simulink model "InvPendu_RBF"  (R2020b)
settings: Solver=VariableStepAuto  StartTime=0.0  StopTime=50  RelTol=1e-3
settings Model: Creator=lenovo  LastModifiedBy=lenovo

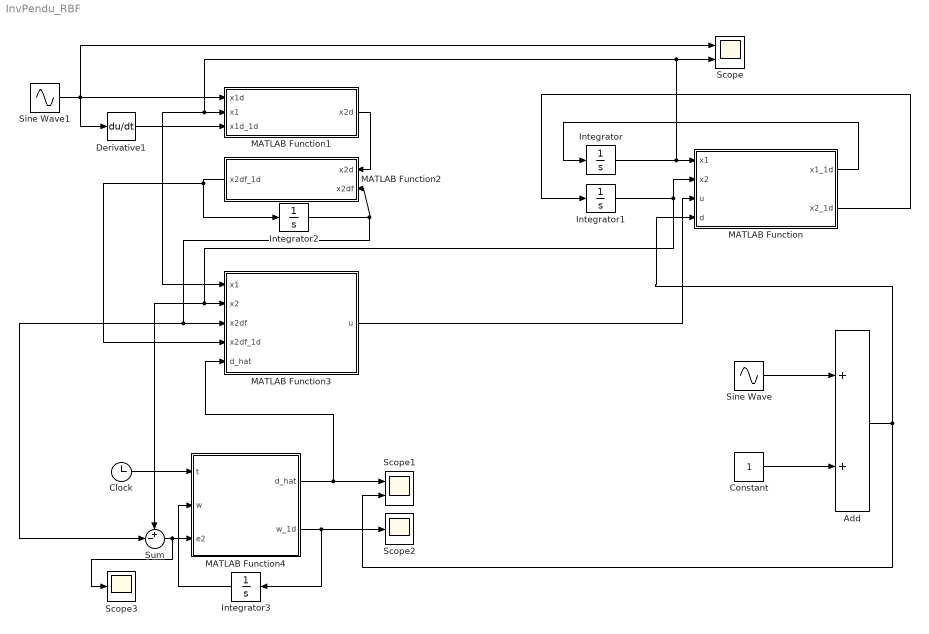
== system InvPendu_RBF ==
  Add : Sum
  Clock : Clock
  Constant : Constant
  Derivative1 : Derivative
  Integrator{,1..3} (4 alike) : Integrator
  MATLAB Function : MATLAB Function  TreatAsAtomicUnit=on
  MATLAB Function1 : MATLAB Function  TreatAsAtomicUnit=on
  MATLAB Function2 : MATLAB Function  TreatAsAtomicUnit=on
  MATLAB Function3 : MATLAB Function  TreatAsAtomicUnit=on
  MATLAB Function4 : MATLAB Function  TreatAsAtomicUnit=on
  Scope : Scope  NumInputPorts=2
  Scope1 : Scope  NumInputPorts=2
  Scope2 : Scope
  Scope3 : Scope
  Sine Wave : Sin  SampleTime=0
  Sine Wave1 : Sin  SampleTime=0
  Sum : Sum  Inputs=+-|
  wires:
  MATLAB Function/1(x1_1d) -> Integrator/1
  Integrator/1 -> Scope/2, MATLAB Function3/1(x1), MATLAB Function1/2(x1), MATLAB Function/1(x1)
  MATLAB Function/2(x2_1d) -> Integrator1/1
  Add/1 -> MATLAB Function/4(d), Scope1/2
  MATLAB Function3/1(u) -> MATLAB Function/3(u)
  Constant/1 -> Add/2
  MATLAB Function2/1(x2df_1d) -> MATLAB Function3/4(x2df_1d), Integrator2/1
  Integrator2/1 -> MATLAB Function3/3(x2df), Sum/2, MATLAB Function2/2(x2df)
  Derivative1/1 -> MATLAB Function1/3(x1d_1d)
  MATLAB Function1/1(x2d) -> MATLAB Function2/1(x2d)
  Sine Wave1/1 -> Derivative1/1, Scope/1, MATLAB Function1/1(x1d)
  Sine Wave/1 -> Add/1
  MATLAB Function4/1(d_hat) -> MATLAB Function3/5(d_hat), Scope1/1
  Integrator1/1 -> Sum/1, MATLAB Function3/2(x2), MATLAB Function/2(x2)
  Clock/1 -> MATLAB Function4/1(t)
  MATLAB Function4/2(w_1d) -> Scope2/1, Integrator3/1
  Integrator3/1 -> MATLAB Function4/2(w)
  Sum/1 -> Scope3/1, MATLAB Function4/3(e2)

== matlab function InvPendu_RBF/MATLAB Function1 ==
  data: x1d input; x1 input; x1d_1d input; x2d output
function x2d = Controller1(x1d,x1,x1d_1d)
    k1 = 5;
    
    e1 = x1 - x1d;
    
x2d = -k1*e1 + x1d_1d;

== matlab function InvPendu_RBF/MATLAB Function ==
  data: x1 input; x2 input; u input; x1_1d output; d input; x2_1d output
function [x1_1d,x2_1d] = InvPendu_Model(x1,x2,u,d)
    M = 10;
    m = 2;
    g = 10;
    L = 5;

x1_1d = x2;
x2_1d = ((M+m)*g*sin(x1))/((M+m*(sin(x1))^2)*L) - (m*L*sin(x1)*cos(x1)*x2^2)/((M+m*(sin(x1))^2)*L) - cos(x1)*u + d;

== matlab function InvPendu_RBF/MATLAB Function2 ==
  data: x2d input; x2df_1d output; x2df input
function x2df_1d = Filter(x2d,x2df)
    tau = 0.1;
    
x2df_1d = (x2d-x2df)/tau;

== matlab function InvPendu_RBF/MATLAB Function3 ==
  data: x1 input; u output; x2 input; x2df input; x2df_1d input; d_hat input
function u = Controller2(x1,x2,x2df,x2df_1d,d_hat)
    M = 10;
    m = 2;
    L = 5;
    k2 = 5;
    g = 10;
    
    e2 = x2 - x2df;
%     temp1 = ((M+m)*g*sin(x1))/((M+m*(sin(x1))^2)*L);
%     temp2 = (m*L*sin(x1)*cos(x1)*x2^2)/((M+m*(sin(x1))^2)*L);

% u = (k2*e2)/(cos(x1)) + (temp1-temp2-x2df_1d)/(cos(x1)) + d_hat/cos(x1);
u = (k2*e2)/(cos(x1)) + (((M+m)*g*sin(x1))/((M+m*(sin(x1))^2)*L)-(m*L*sin(x1)*cos(x1)*x2^2)/((M+m*(sin(x1))^2)*L)-x2df_1d)/(cos(x1)) + d_hat/cos(x1);

== matlab function InvPendu_RBF/MATLAB Function4 ==
  data: d_hat output size=1; t input size=1; w_1d output size=[11,1]; w input size=[11,1]; e2 input size=1
function [d_hat,w_1d]= RBFNN(t,w,e2)
    k3 = 5;
    s = zeros(11,1);
    c = [-1,-0.8,-0.6,-0.4,-0.2,0,0.2,0.4,0.6,0.8,1];
    b = [1,1,1,1,1,1,1,1,1,1,1];
    for i = 1:1:11
        s(i) = exp((-(t-c(i))^2)/(b(i)^2));
    end
   
   y = w'*s;
   
   
   w_1d = -k3*w + s*e2;
   d_hat = y;
